simulink model "DigitalFilterExample"  (R2017a)
settings: Solver=VariableStepAuto  StartTime=0.0  StopTime=.4  MaxStep=1e-4  RelTol=1e-3
libraries: simulink x2, simulink_extras x1
settings Model: Creator=erich  LastModifiedBy=erich

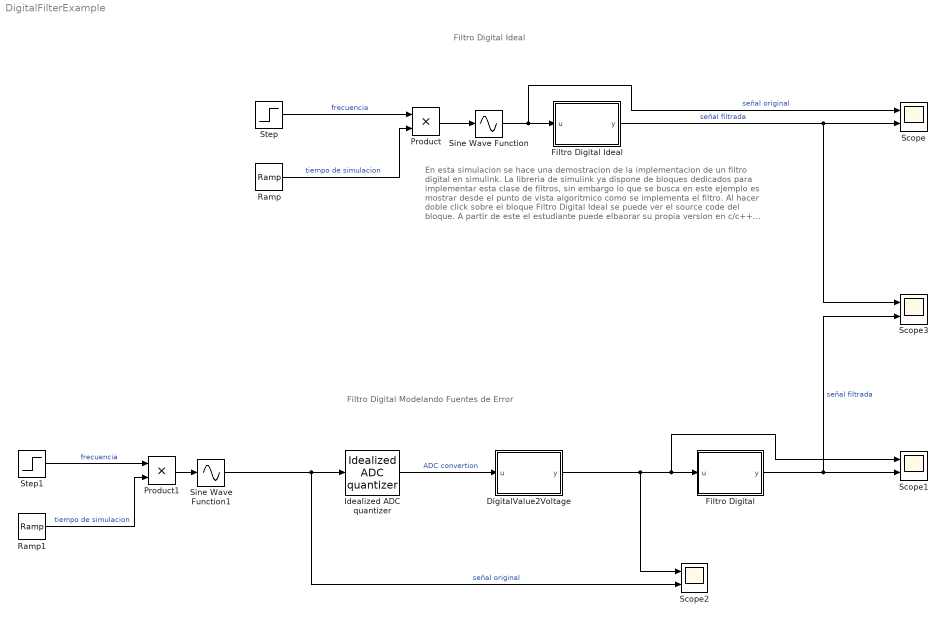
== system DigitalFilterExample ==
  note: Filtro Digital Ideal
  note: En esta simulacion se hace una demostracion de la implementacion de
      | un filtro digital en simulink.
      | La libreria de simulink ya dispone de bloques dedicados para implementar
      | esta clase de filtros, sin embargo lo que se busca en este ejemplo es mostrar
      | desde el punto de vista algoritmico como se implementa el filtro. Al
      | hacer doble click sobre el bloque Filtro Digital Ideal se puede ver el source
      | code del bloque. A partir de este el estudiante puede elbaorar su propia
      | version en c/c++ para implementarlo en un sistema embebido.
      |
      | el tiempo de muestreo del bloque fcn se modifica haciendo click derecho y
      | accediendo a la opcion subsystem properties. Alli, en la parte inferior de
      | se puede modificar el sampling time.
  note: Filtro Digital Modelando Fuentes de Error
  DigitalValue2Voltage : MATLAB Function  TreatAsAtomicUnit=on  SystemSampleTime=1e-3
  Filtro Digital : MATLAB Function  TreatAsAtomicUnit=on  SystemSampleTime=1e-3
  Filtro Digital Ideal : MATLAB Function  TreatAsAtomicUnit=on  SystemSampleTime=1e-3
  Idealized ADC quantizer : simulink_extras/Additional Discrete/Idealized ADC quantizer  NumberOfConverterBits=10  Vmin=-5  Vmax=5  OutputDataType=double  OutputNegativeValues=on
      settings: SourceProductName=Simulink
  Product : Product
  Product1 : Product
  Ramp : simulink/Sources/Ramp  slope=1  start=0  X0=0
  Ramp1 : simulink/Sources/Ramp  slope=1  start=0  X0=0
  Scope{,1..3} (4 alike) : Scope  NumInputPorts=2
  Sine Wave Function : Sin  TimeSource=Use external signal  Amplitude=2  SampleTime=0
  Sine Wave Function1 : Sin  TimeSource=Use external signal  Amplitude=2  SampleTime=0
  Step : Step  Time=.2  Before=2*pi*55  After=2*pi*100  SampleTime=0
  Step1 : Step  Time=.2  Before=2*pi*55  After=2*pi*100  SampleTime=0
  wires:
  Sine Wave Function/1 -> Scope/1, Filtro Digital Ideal/1(u)  "señal original"
  Filtro Digital Ideal/1(y) -> Scope3/1, Scope/2  "señal filtrada"
  Product/1 -> Sine Wave Function/1
  Ramp/1 -> Product/2  "tiempo de simulacion"
  Step/1 -> Product/1  "frecuencia"
  Step1/1 -> Product1/1  "frecuencia"
  Ramp1/1 -> Product1/2  "tiempo de simulacion"
  Product1/1 -> Sine Wave Function1/1
  Filtro Digital/1(y) -> Scope3/2, Scope1/2  "señal filtrada"
  Sine Wave Function1/1 -> Idealized ADC quantizer/1, Scope2/2  "señal original"
  DigitalValue2Voltage/1(y) -> Scope2/1, Filtro Digital/1(u), Scope1/1
  Idealized ADC quantizer/1 -> DigitalValue2Voltage/1(u)  "ADC convertion"

== matlab function DigitalFilterExample/Filtro Digital ==
  data: u input; y output
function y = fcn(u)


% coeficientes del filtro fir
FIR = [-0.00128380297866020 -0.00132399486984157 0.000874051194962120 0.00518832470467140 0.00810033142850478 0.00521435647752571 -0.00383759191001733 -0.0130617913066840 -0.0144823190219763 -0.00642101723421765 0.00313914084679193 0.00398182413302851 -0.00377232760690022 -0.00607061854849465 0.0117264683573292 0.0446289841467845 0.0629963601398514 0.0346660062390859 -0.0407342672859202 -0.118248982958290 -0.134988177907574 -0.0618228722171959 0.0645157002731517 0.161472913942402 0.161472913942402 0.0645157002731517 -0.0618228722171959 -0.134988177907574 -0.118248982958290 -0.0407342672859202 0.0346660062390859 0.0629963601398514 0.0446289841467845 0.0117264683573292 -0.00607061854849465 -0.00377232760690022 0.00398182413302851 0.00313914084679193 -0.00642101723421765 -0.0144823190219763 -0.0130617913066840 -0.00383759191001733 0.00521435647752571 0.00810033142850478 0.00518832470467140 0.000874051194962120 -0.00132399486984157 -0.00128380297866020];

coder.extrinsic('round');

FIR = round(FIR, 3); % cuando el procesador no posee la arquitectura necesaria para guardar todos los decimales

% de un numero, este es truncado. Es puede generar desviaciones del
% comportamiento esperado si los parametros poseen mucha sensibilidad.
% en este caso se intenta modelar este efecto.

% variable persistente, se guardan los valores de la variable window entre
% despues de salir de este scope
persistent window2;

% cuando se ejecuta por primera vez, window sera una variable nula.
% este condicional permite inicializar el valor de window la primera vez
% que se ejecuta el codigo.
if isempty(window2)
    window2 = zeros(1,length(FIR));
end

% se hace un shift de los valores leidos de la señal de entrada.
window2 = [u window2(1:end-1)];

% se hace el calculo del filtro fir se pone el resultado  a la salida
% de  este bloque.
y = FIR*window2';

== matlab function DigitalFilterExample/Filtro Digital Ideal ==
  data: u input; y output
function y = fcn(u)


% coeficientes del filtro fir
FIR = [-0.00128380297866020 -0.00132399486984157 0.000874051194962120 0.00518832470467140 0.00810033142850478 0.00521435647752571 -0.00383759191001733 -0.0130617913066840 -0.0144823190219763 -0.00642101723421765 0.00313914084679193 0.00398182413302851 -0.00377232760690022 -0.00607061854849465 0.0117264683573292 0.0446289841467845 0.0629963601398514 0.0346660062390859 -0.0407342672859202 -0.118248982958290 -0.134988177907574 -0.0618228722171959 0.0645157002731517 0.161472913942402 0.161472913942402 0.0645157002731517 -0.0618228722171959 -0.134988177907574 -0.118248982958290 -0.0407342672859202 0.0346660062390859 0.0629963601398514 0.0446289841467845 0.0117264683573292 -0.00607061854849465 -0.00377232760690022 0.00398182413302851 0.00313914084679193 -0.00642101723421765 -0.0144823190219763 -0.0130617913066840 -0.00383759191001733 0.00521435647752571 0.00810033142850478 0.00518832470467140 0.000874051194962120 -0.00132399486984157 -0.00128380297866020];

% variable persistente, se guardan los valores de la variable window entre
% despues de salir de este scope
persistent window;

% cuando se ejecuta por primera vez, window sera una variable nula.
% este condicional permite inicializar el valor de window la primera vez
% que se ejecuta el codigo.
if isempty(window)
    window = zeros(1,length(FIR));
end

% se hace un shift de los valores leidos de la señal de entrada.
window = [u window(1:end-1)];

% se hace el calculo del filtro fir se pone el resultado  a la salida
% de  este bloque.
y = FIR*window';

== matlab function DigitalFilterExample/DigitalValue2Voltage ==
  data: u input; y output
function y = fcn(u)


bits = 9; % resolucion del adc (10 bits  en este caso)
% sin embargo, debido a que se deben representar tambien valores negativos
% entonces la resolucion se reduce a la mitad. por eso no se pone 2^10 sino
% que se tienen 2^9 valores para representar valores positivos y 2^9
% valores para representar valores negativos.
ref = 5; % tension de referencia del ADC 

y = u/2^(bits)*ref;
